simulink model "motor_tune"  (Simulink 8.2)
settings: Solver=ode45  StartTime=0.0  StopTime=inf  RelTol=1e-3
values from neighbouring files (symbols this model uses):
  s = evalin('base','s')    [GUI_MT218.m]
undefined symbols (not defined in the file or in its folder): TS_boat
undefined symbols (not defined in the file): controller
libraries: simulink x2
settings Model: Creator=Andries  LastModifiedBy=mgodjevac

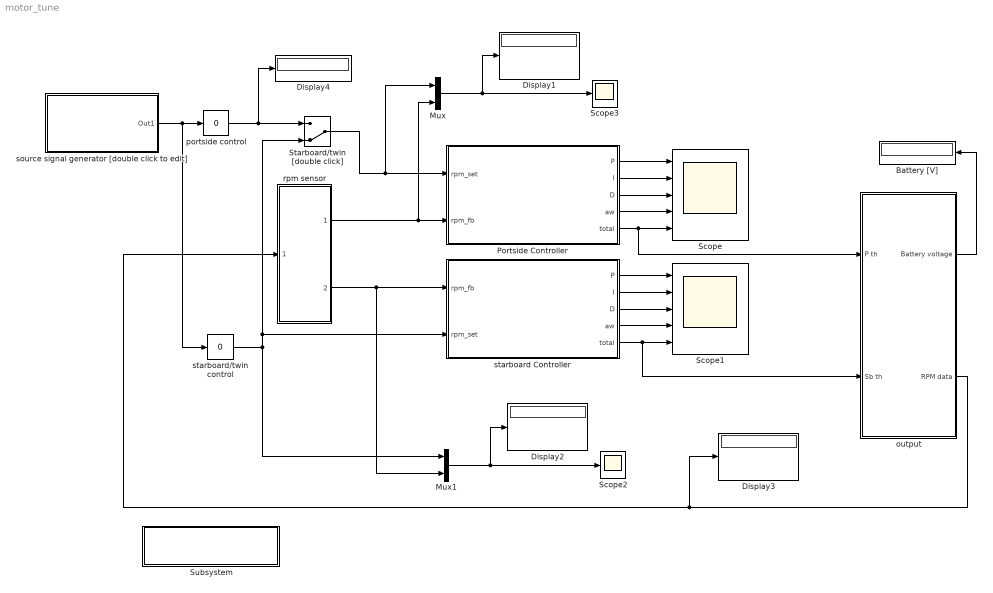
== system motor_tune ==
  Battery [V] : Display
  Display{1..4} (4 alike) : Display
  Mux : Mux  Inputs=2
  Mux1 : Mux  Inputs=2
  Portside Controller : Subsystem  mask{P=controller.PP, I=controller.PI, D=controller.PD, P_aw=controller.PPaw}
      mask help: Controller setting for Starboard engine
  Scope : Scope  NumInputPorts=5
      settings: YMin=-5~-5~-5~-5~-5  YMax=5~5~5~5~5
  Scope1 : Scope  NumInputPorts=5
      settings: YMin=-5~-5~-5~-5~-5  YMax=5~5~5~5~5  SaveName=ScopeData2
  Scope2 : Scope
      settings: SaveName=ScopeData3
  Scope3 : Scope
      settings: YMin=-0  YMax=14  SaveName=ScopeData4
  Starboard/twin [double click] : ManualSwitch  CurrentSetting=0
  Subsystem : Subsystem
      mask Display:
      | if evalin('base','exist(''boat'')');
      |     set_param(gcb,'BackgroundColor','Green')
      |     disp(['connected to: ',evalin('base','boat.name')]);
      | else
      |     disp('no boat connected')
      |     set_param(gcb,'BackgroundColor','Red')
      |     color('red')
      | end
  output : Subsystem
  portside control : simulink/Math Operations/Slider Gain  low=-1100  gain=0  high=1500
  rpm sensor : Subsystem  mask{n_p=controller.Prpm, n_sb=controller.STrpm}
      mask prompts: n_p "Amount of holes in portside RPM sensor disc"; n_sb "Amount of holes in portside RPM sensor disc"
      mask Display:
      | port_label('output', 1, 'Ps RPM')
      | port_label('output', 2, 'SBs RPM')
  source signal generator [double click to edit] : Subsystem  mask{sw=constant value, freq=.5}
      mask prompts: sw "signal type"; freq "frequency"
      mask TypeOptions sw: constant value | sine wave
      mask Display:
      | if sw == 1
      |     disp('constant value')
      | else
      |     disp(['sine wave, freq: ',num2str(freq)])
      | end
  starboard Controller : Subsystem  mask{P=controller.STP, I=controller.STI, D=controller.STD, P_aw=controller.STPaw}
      mask help: Controller setting for Starboard engine
  starboard/twin control : simulink/Math Operations/Slider Gain  low=-1100  gain=0  high=1500
  wires:
  source signal generator [double click to edit]/1(Out1) -> portside control/1, starboard/twin control/1
  rpm sensor/1(portside rpm) -> Portside Controller/2(rpm_fb), Mux/2
  rpm sensor/2(starboard side rpm) -> starboard Controller/1(rpm_fb), Mux1/2
  starboard Controller/5(total) -> Scope1/5, output/2(Sb th)
  Portside Controller/5(total) -> Scope/5, output/1(P th)
  Portside Controller/1(" P") -> Scope/1
  Portside Controller/2(I) -> Scope/2
  Portside Controller/3(D) -> Scope/3
  Portside Controller/4(aw) -> Scope/4
  starboard Controller/4(aw) -> Scope1/4
  starboard Controller/3(D) -> Scope1/3
  starboard Controller/2(I) -> Scope1/2
  starboard Controller/1(" P") -> Scope1/1
  Starboard/twin [double click]/1 -> Portside Controller/1(rpm_set), Mux/1
  portside control/1 -> Starboard/twin [double click]/1, Display4/1
  Mux/1 -> Scope3/1, Display1/1
  output/2(RPM data) -> Display3/1, rpm sensor/1(RPM data)
  Mux1/1 -> Display2/1, Scope2/1
  starboard/twin control/1 -> Mux1/1, Starboard/twin [double click]/2, starboard Controller/2(rpm_set)
  output/1(Battery voltage) -> Battery [V]/1

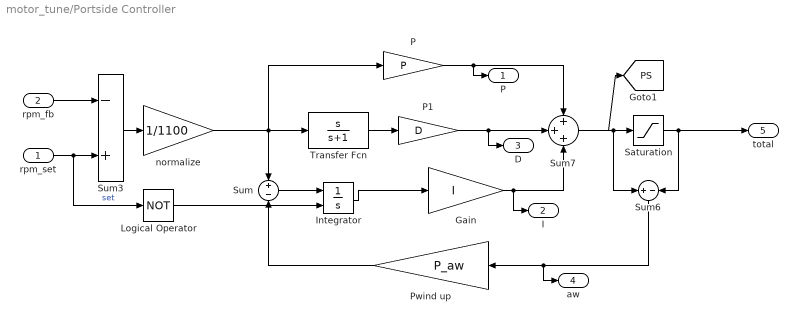
== system motor_tune/Portside Controller ==
  rpm_set : Inport
  rpm_fb : Inport  Port=2
  Gain : Gain  Gain=I  SaturateOnIntegerOverflow=on  OutDataTypeStr=Inherit: Same as input  ParamDataTypeStr=Inherit: Same as input
  Integrator : Integrator  ExternalReset=level
  Logical Operator : Logic  Operator=NOT  AllPortsSameDT=off  OutDataTypeStr=boolean
  P : Gain  Gain=P  SaturateOnIntegerOverflow=on  OutDataTypeStr=Inherit: Same as input  ParamDataTypeStr=Inherit: Same as input
  P1 : Gain  Gain=D  SaturateOnIntegerOverflow=on  OutDataTypeStr=Inherit: Same as input  ParamDataTypeStr=Inherit: Same as input
  Pwind up : Gain  Gain=P_aw  SaturateOnIntegerOverflow=on  OutDataTypeStr=Inherit: Same as input  ParamDataTypeStr=Inherit: Same as input
  Saturation : Saturate  UpperLimit=1  LowerLimit=-1
  Sum : Sum  Inputs=+|-  SaturateOnIntegerOverflow=on
  Sum3 : Sum  Inputs=-+  SaturateOnIntegerOverflow=on  InputSameDT=on  OutDataTypeStr=Inherit: Same as first input
  Sum6 : Sum  Inputs=+-  SaturateOnIntegerOverflow=on  InputSameDT=on  OutDataTypeStr=Inherit: Same as first input
  Sum7 : Sum  Inputs=+++  SaturateOnIntegerOverflow=on  InputSameDT=on  OutDataTypeStr=Inherit: Same as first input
  Transfer Fcn : TransferFcn  Numerator=[1 0]  Denominator=[1 1]
  normalize : Gain  Gain=1/1100
  " P" : Outport
  I : Outport  Port=2
  D : Outport  Port=3
  aw : Outport  Port=4
  total : Outport  Port=5
  tag scope: PS=global
  wires:
  rpm_fb/1 -> Sum3/1
  Sum/1 -> Integrator/1
  Pwind up/1 -> Sum/2
  Sum6/1 -> Pwind up/1, aw/1
  Sum7/1 -> Sum6/1, Saturation/1, [PS]
  Saturation/1 -> Sum6/2, total/1
  P/1 -> Sum7/1, " P"/1
  Sum3/1 -> normalize/1
  Integrator/1 -> Gain/1
  Gain/1 -> Sum7/3, I/1
  P1/1 -> Sum7/2, D/1
  Transfer Fcn/1 -> P1/1
  rpm_set/1 -> Sum3/2, Logical Operator/1  "set"
  normalize/1 -> Sum/1, P/1, Transfer Fcn/1
  Logical Operator/1 -> Integrator/2

== system motor_tune/Subsystem ==

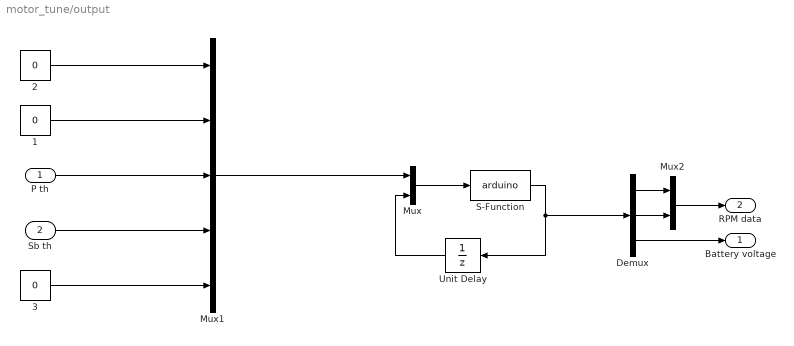
== system motor_tune/output ==
  P th : Inport
  Sb th : Inport  Port=2
  1 : Constant  Value=0
  2 : Constant  Value=0
  3 : Constant  Value=0
  Demux : Demux  Outputs=3
  Mux : Mux  Inputs=2
  Mux1 : Mux  Inputs=5
  Mux2 : Mux  Inputs=2
  S-Function : S-Function  FunctionName=arduino  Parameters=TS_boat,s  EnableBusSupport=off
  Unit Delay : UnitDelay  SampleTime=-1
  Battery voltage : Outport
  RPM data : Outport  Port=2
  wires:
  Mux1/1 -> Mux/1
  1/1 -> Mux1/2
  3/1 -> Mux1/5
  2/1 -> Mux1/1
  P th/1 -> Mux1/3
  Sb th/1 -> Mux1/4
  Mux/1 -> S-Function/1
  Unit Delay/1 -> Mux/2
  S-Function/1 -> Demux/1, Unit Delay/1
  Demux/1 -> Mux2/1
  Demux/2 -> Mux2/2
  Mux2/1 -> RPM data/1
  Demux/3 -> Battery voltage/1

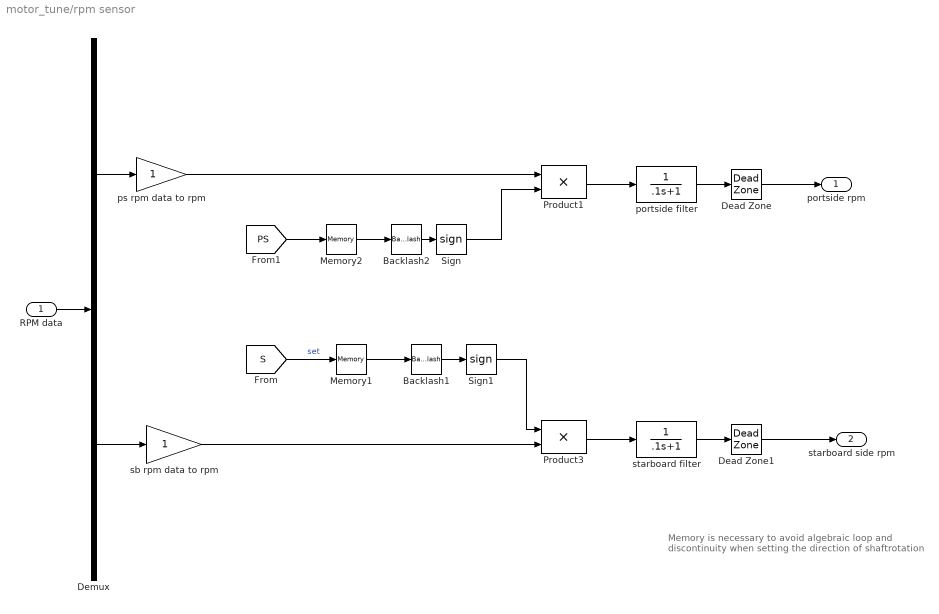
== system motor_tune/rpm sensor ==
  note: Memory is necessary to avoid algebraic loop
      |  and discontinuity when setting the
      |  direction of shaftrotation
  RPM data : Inport
  " sb rpm data to rpm" : Gain
  Backlash1 : Backlash  BacklashWidth=.1
  Backlash2 : Backlash  BacklashWidth=.1
  Dead Zone : DeadZone  SaturateOnIntegerOverflow=on
  Dead Zone1 : DeadZone  SaturateOnIntegerOverflow=on
  Demux : Demux  Outputs=2
  Memory1 : Memory  X0=1
  Memory2 : Memory  X0=1
  Product1 : Product  SaturateOnIntegerOverflow=on  InputSameDT=on  OutDataTypeStr=Inherit: Same as first input
  Product3 : Product  SaturateOnIntegerOverflow=on  InputSameDT=on  OutDataTypeStr=Inherit: Same as first input
  Sign : Signum
  Sign1 : Signum
  portside filter : TransferFcn  Denominator=[.1 1]
  ps rpm data to rpm : Gain
  starboard filter : TransferFcn  Denominator=[.1 1]
  portside rpm : Outport
  starboard side rpm : Outport  Port=2
  wires:
  RPM data/1 -> Demux/1
  Memory2/1 -> Backlash2/1
  Backlash2/1 -> Sign/1
  Product3/1 -> starboard filter/1
  Sign/1 -> Product1/2
  [PS] -> Memory2/1
  Memory1/1 -> Backlash1/1
  Backlash1/1 -> Sign1/1
  [S] -> Memory1/1  "set"
  Sign1/1 -> Product3/1
  Dead Zone/1 -> portside rpm/1
  Dead Zone1/1 -> starboard side rpm/1
  Demux/1 -> ps rpm data to rpm/1
  Demux/2 -> " sb rpm data to rpm"/1
  Product1/1 -> portside filter/1
  " sb rpm data to rpm"/1 -> Product3/2
  starboard filter/1 -> Dead Zone1/1
  ps rpm data to rpm/1 -> Product1/1
  portside filter/1 -> Dead Zone/1

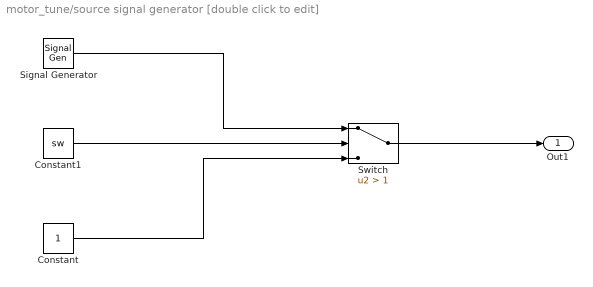
== system motor_tune/source signal generator [double click to edit] ==
  Constant : Constant
  Constant1 : Constant  Value=sw
  Signal Generator : SignalGenerator  Frequency=freq  Units=rad/sec
  Switch : Switch  Criteria=u2 > Threshold  Threshold=1
  Out1 : Outport
  wires:
  Switch/1 -> Out1/1
  Constant1/1 -> Switch/2
  Signal Generator/1 -> Switch/1
  Constant/1 -> Switch/3

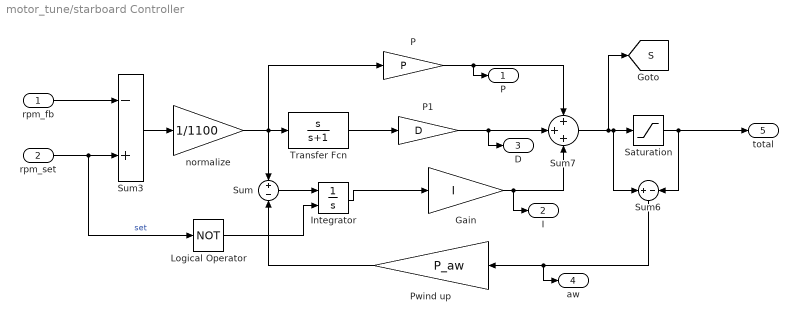
== system motor_tune/starboard Controller ==
  rpm_fb : Inport
  rpm_set : Inport  Port=2
  Gain : Gain  Gain=I  SaturateOnIntegerOverflow=on  OutDataTypeStr=Inherit: Same as input  ParamDataTypeStr=Inherit: Same as input
  Integrator : Integrator  ExternalReset=level
  Logical Operator : Logic  Operator=NOT  AllPortsSameDT=off  OutDataTypeStr=boolean
  P : Gain  Gain=P  SaturateOnIntegerOverflow=on  OutDataTypeStr=Inherit: Same as input  ParamDataTypeStr=Inherit: Same as input
  P1 : Gain  Gain=D  SaturateOnIntegerOverflow=on  OutDataTypeStr=Inherit: Same as input  ParamDataTypeStr=Inherit: Same as input
  Pwind up : Gain  Gain=P_aw  SaturateOnIntegerOverflow=on  OutDataTypeStr=Inherit: Same as input  ParamDataTypeStr=Inherit: Same as input
  Saturation : Saturate  UpperLimit=1  LowerLimit=-1
  Sum : Sum  Inputs=+|-  SaturateOnIntegerOverflow=on
  Sum3 : Sum  Inputs=-+  SaturateOnIntegerOverflow=on  InputSameDT=on  OutDataTypeStr=Inherit: Same as first input
  Sum6 : Sum  Inputs=+-  SaturateOnIntegerOverflow=on  InputSameDT=on  OutDataTypeStr=Inherit: Same as first input
  Sum7 : Sum  Inputs=+++  SaturateOnIntegerOverflow=on  InputSameDT=on  OutDataTypeStr=Inherit: Same as first input
  Transfer Fcn : TransferFcn  Numerator=[1 0]  Denominator=[1 1]
  normalize : Gain  Gain=1/1100
  " P" : Outport
  I : Outport  Port=2
  D : Outport  Port=3
  aw : Outport  Port=4
  total : Outport  Port=5
  tag scope: S=global
  wires:
  Transfer Fcn/1 -> P1/1
  P1/1 -> D/1, Sum7/2
  Gain/1 -> I/1, Sum7/3
  Integrator/1 -> Gain/1
  Sum3/1 -> normalize/1
  P/1 -> " P"/1, Sum7/1
  Saturation/1 -> Sum6/2, total/1
  Sum7/1 -> Saturation/1, Sum6/1, [S]
  Sum6/1 -> aw/1, Pwind up/1
  Pwind up/1 -> Sum/2
  Sum/1 -> Integrator/1
  rpm_fb/1 -> Sum3/1
  rpm_set/1 -> Sum3/2, Logical Operator/1  "set"
  normalize/1 -> P/1, Sum/1, Transfer Fcn/1
  Logical Operator/1 -> Integrator/2
